simulink model "Test"  (R2021a)
settings: Solver=FixedStepAuto  StartTime=0.0  StopTime=0.1  FixedStep=1/44100  RelTol=1e-3
libraries: dspsnks4 x1
settings Model: Creator=ZZDDD  LastModifiedBy=ZZDDD
settings SolverCC: AlgebraicLoopSolver=TrustRegion
settings DataIOCC: LimitDataPoints=on  SaveOutput=off  SaveTime=off
settings OptimizationCC: BlockReduction=off  BooleanDataType=off  LifeSpan=inf
settings DebuggingCC: SaveWithParameterizedLinksMsg=none  UnderspecifiedInitializationDetection=Classic  MergeDetectMultiDrivingBlocksExec=none  SignalResolutionControl=TryResolveAllWithWarning  AllowSymbolicDim=off  SFUnexpectedBacktrackingDiag=warning  SFNoUnconditionalDefaultTransitionDiag=warning  SFExecutionAtInitializationDiag=none  SFMachineParentedDataDiag=warning  ArithmeticOperatorsInVariantConditions=warning
settings HardwareCC: TargetUnknown=on
settings SFSimCC: SimUseLocalCustomCode=off  CustomCodeUndefinedFunction=UseInterfaceOnly
settings RTWCC: RTWUseLocalCustomCode=off
settings CodeAppCC: StateflowObjectComments=on
settings GRTTargetCC: TargetLangStandard=C89/C90 (ANSI)

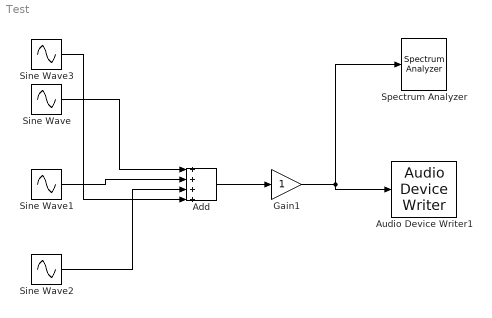
== system Test ==
  Add : Sum  Inputs=++++
  Audio Device Writer1 : dspsnks4/Audio Device Writer  Driver=DirectSound  Device=Default  InheritSampleRate=on  SampleRate=44100  BitDepth=16-bit integer  BufferSize=4096  NumBuffers=10  DefaultOutputChannelMapping=on  OutputChannelMapping=1:2  OutputNumUnderrunSamples=off  DriverIdx=1  DeviceWarnFlag=''
  Gain1 : Gain  OutDataTypeStr=Inherit: Same as input
  Sine Wave : Sin  Amplitude=0.8  Frequency=440 * 2 * pi  SampleTime=1/44100
  Sine Wave1 : Sin  Amplitude=0.4  Frequency=440 * 2 * pi * 2  SampleTime=1/44100
  Sine Wave2 : Sin  Amplitude=0.2  Frequency=440 * 2 * pi * 3  SampleTime=1/44100
  Sine Wave3 : Sin  Amplitude=1.6  Frequency=440 * 2 * pi / 2  SampleTime=1/44100
  Spectrum Analyzer : SpectrumAnalyzer
  wires:
  Gain1/1 -> Audio Device Writer1/1, Spectrum Analyzer/1
  Sine Wave/1 -> Add/1
  Sine Wave1/1 -> Add/2
  Add/1 -> Gain1/1
  Sine Wave2/1 -> Add/3
  Sine Wave3/1 -> Add/4
